simulink model "Adaptive_CT_ur10v"  (R2021b)
settings: Solver=VariableStepAuto  StartTime=0.0  StopTime=15  FixedStep=1e-4  RelTol=1e1
values from neighbouring files (symbols this model uses):
  Kp = [100 0 0 0 0 0 0 250 0 0 0 0 ... (36 elements, 6x6)]    [ACT_workspace.mat]    (also in GuadagniControllore.m = 100 * diag([1 1 2 4 5 5]))
  Kv = [100 0 0 0 0 0 0 100 0 0 0 0 ... (36 elements, 6x6)]    [ACT_workspace.mat]    (also in GuadagniControllore.m = 100 * diag([1 1 3 3 5 5]))
  l1 = 0.1273    [ACT_workspace.mat]
  l2 = -0.612    [ACT_workspace.mat]
  l3 = -0.5723    [ACT_workspace.mat]
  l4 = 0.1639    [ACT_workspace.mat]
  l5 = 0.1157    [ACT_workspace.mat]
  l6 = 0.0922    [ACT_workspace.mat]
  m1 = 7.1    [ACT_workspace.mat]
  m2 = 12.7    [ACT_workspace.mat]
  m3 = 4.27    [ACT_workspace.mat]
  m4 = 2    [ACT_workspace.mat]
  m5 = 2    [ACT_workspace.mat]
  m6 = 0.365    [ACT_workspace.mat]
  q0 = [0 0 0 0 0 0]    [ACT_workspace.mat]
  r = 0.02    [ACT_workspace.mat]
undefined symbols (not defined in the file or in its folder): B, Spline
libraries: roblocks x2, robotcorelib x1, simulink x1
(part 3 of 20)

== matlab function Adaptive_CT_ur10v/CT control/Subsystem/Regressor ==
  data: q input; Y output; qd input; qdd input
function Y = Regressor(q, qd, qdd)
%#codegen

q2 = q(2);
q3 = q(3);
q4 = q(4);
q5 = q(5);
q6 = q(6);
qd1 = qd(1);
qd2 = qd(2);
qd3 = qd(3);
qd4 = qd(4);
qd5 = qd(5);
qd6 = qd(6);
qdd1 = qdd(1);
qdd2 = qdd(2);
qdd3 = qdd(3);
qdd4 = qdd(4);
qdd5 = qdd(5);
qdd6 = qdd(6);


%    This function was generated by the Symbolic Math Toolbox version 9.0.
%    07-Jul-2022 14:08:40

t2 = cos(q2);
t3 = cos(q3);
t4 = cos(q4);
t5 = cos(q5);
t6 = sin(q2);
t7 = sin(q3);
t8 = sin(q4);
t9 = sin(q5);
t10 = q2+q3;
t11 = q2+q5;
t12 = q3+q4;
t13 = q4+q5;
t14 = qdd2+qdd3;
t15 = q2.*2.0;
t16 = q3.*2.0;
t17 = q4.*2.0;
t18 = q5.*2.0;
t19 = qd1.^2;
t20 = qd2.^2;
t21 = qd3.^2;
t22 = qd4.^2;
t23 = qd5.^2;
t41 = -q5;
t51 = qdd1./2.0;
t52 = qdd2./2.0;
t53 = qdd1./4.0;
t54 = qdd3./2.0;
t55 = qdd4./2.0;
t117 = qdd2.*9.22e-2;
t118 = qdd3.*9.22e-2;
t119 = qdd4.*9.22e-2;
t302 = qdd3.*3.451642e-1;
t397 = qdd3.*3.4091378e-1;
t401 = qdd4.*1.338649e-2;
t402 = qdd4.*1.763691e-2;
t466 = qdd2.*3.2752729e-1;
t467 = qdd3.*3.2752729e-1;
t530 = qdd2.*7.0207129e-1;
t24 = cos(t15);
t25 = cos(t18);
t26 = t2.^2;
t27 = sin(t15);
t28 = sin(t18);
t29 = cos(t10);
t30 = cos(t11);
t31 = cos(t12);
t32 = cos(t13);
t33 = q4+t10;
t34 = q5+t10;
t35 = q5+t12;
t36 = qdd4+t14;
t37 = sin(t10);
t38 = sin(t11);
t39 = sin(t12);
t40 = sin(t13);
t42 = -t18;
t46 = t10+t13;
t50 = q2+t10;
t61 = q2+t41;
t62 = q4+t41;
t63 = t10.*2.0;
t66 = t10+t41;
t67 = t12+t41;
t94 = qd1.*qd2.*t2.*t6.*2.0;
t143 = qdd1.*t5.*3.278e-1;
t145 = qdd2.*t8.*1.1446;
t146 = qdd3.*t8.*1.1446;
t156 = qd2.*qd4.*t4.*1.1446;
t157 = qd3.*qd4.*t4.*1.1446;
t158 = qd1.*qd5.*t9.*3.278e-1;
t178 = qdd2.*t5.*1.157e-1;
t179 = qdd3.*t5.*1.157e-1;
t180 = qdd4.*t5.*1.157e-1;
t181 = qdd5.*t5.*1.157e-1;
t184 = qdd4.*t8.*5.723e-1;
t211 = t2.*6.00372;
t248 = t4.*t22.*5.723e-1;
t251 = t9.*t23.*1.157e-1;
t252 = t9.*t19.*1.639e-1;
t348 = qdd1.*t6.*1.003068e-1;
t349 = qdd2.*t6.*1.003068e-1;
t379 = qdd2.*t3.*7.004952e-1;
t380 = qdd1.*t3.*3.502476e-1;
t381 = qdd2.*t3.*3.502476e-1;
t382 = qdd3.*t3.*3.502476e-1;
t418 = t2.*t20.*1.003068e-1;
t422 = qd2.*qd3.*t7.*7.004952e-1;
t423 = qd1.*qd3.*t7.*3.502476e-1;
t454 = qdd5.*t5.*1.066754e-2;
t463 = qdd2.*t8.*1.3243022e-1;
t464 = qdd3.*t8.*1.3243022e-1;
t479 = t7.*t20.*3.502476e-1;
t480 = t7.*t21.*3.502476e-1;
t481 = t7.*t19.*1.751238e-1;
t483 = qd2.*qd3.*t4.*1.3243022e-1;
t484 = qd2.*qd4.*t4.*1.3243022e-1;
t485 = qd3.*qd4.*t4.*1.3243022e-1;
t525 = qdd1.*t8.*6.621511e-2;
t526 = qdd2.*t8.*6.621511e-2;
t527 = qdd3.*t8.*6.621511e-2;
t528 = qdd4.*t8.*6.621511e-2;
t542 = t9.*t23.*1.066754e-2;
t545 = qd1.*qd4.*t4.*6.621511e-2;
t595 = t4.*t20.*6.621511e-2;
t596 = t4.*t21.*6.621511e-2;
t597 = t4.*t22.*6.621511e-2;
t598 = t4.*t19.*3.3107555e-2;
t43 = cos(t33);
t44 = cos(t34);
t45 = cos(t35);
t47 = sin(t33);
t48 = sin(t34);
t49 = sin(t35);
t56 = cos(t50);
t57 = q2+t33;
t58 = sin(t50);
t59 = cos(t46);
t60 = sin(t46);
t64 = cos(t61);
t65 = cos(t62);
t68 = sin(t61);
t69 = sin(t62);
t71 = t13+t34;
t72 = t11+t33;
t74 = qd2.*qd3.*t28;
t75 = qd2.*qd4.*t28;
t76 = qd2.*qd5.*t28;
t77 = qd3.*qd4.*t28;
t78 = qd3.*qd5.*t28;
t79 = qd4.*qd5.*t28;
t80 = cos(t63);
t82 = t10+t33;
t83 = sin(t63);
t84 = cos(t66);
t85 = cos(t67);
t86 = t33+t41;
t87 = t33+t42;
t88 = sin(t66);
t89 = sin(t67);
t95 = t25.*t52;
t96 = t25.*t53;
t97 = t25.*t54;
t98 = t25.*t55;
t103 = t10+t46;
t109 = qdd2.*t25.*(-1.0./2.0);
t110 = qdd3.*t25.*(-1.0./2.0);
t111 = qdd4.*t25.*(-1.0./2.0);
t115 = (qd1.*qd5.*t28)./2.0;
t116 = t17+t63;
t122 = t33+t46;
t126 = (t19.*t27)./2.0;
t127 = (t20.*t28)./2.0;
t128 = (t19.*t28)./4.0;
t129 = (t21.*t28)./2.0;
t130 = (t22.*t28)./2.0;
t133 = t33+t66;
t137 = qdd2.*t39.*(1.53e+2./2.5e+2);
t138 = qdd1.*t38.*(1.53e+2./5.0e+2);
t139 = qdd2.*t38.*(1.53e+2./5.0e+2);
t140 = qdd5.*t38.*(1.53e+2./5.0e+2);
t141 = t46.*2.0;
t152 = t25.*t117;
t153 = t25.*t118;
t154 = t25.*t119;
t182 = -t145;
t183 = -t146;
t190 = qd1.*qd2.*t30.*(1.53e+2./2.5e+2);
t191 = qd1.*qd5.*t30.*(1.53e+2./2.5e+2);
t200 = qdd2.*t25.*(-9.22e-2);
t201 = qdd3.*t25.*(-9.22e-2);
t202 = qdd4.*t25.*(-9.22e-2);
t205 = -t156;
t206 = -t157;
t210 = -t158;
t236 = -t178;
t237 = -t179;
t238 = -t180;
t239 = -t181;
t240 = -t184;
t242 = t20.*t31.*(1.53e+2./2.5e+2);
t243 = t19.*t31.*(1.53e+2./5.0e+2);
t244 = t20.*t30.*(1.53e+2./5.0e+2);
t245 = t23.*t30.*(1.53e+2./5.0e+2);
t256 = -t211;
t263 = qdd2.*t40.*5.723e-1;
t264 = qdd3.*t40.*5.723e-1;
t265 = qdd1.*t40.*2.8615e-1;
t266 = qdd2.*t40.*2.8615e-1;
t267 = qdd3.*t40.*2.8615e-1;
t268 = qdd4.*t40.*2.8615e-1;
t269 = qdd5.*t40.*2.8615e-1;
t279 = -t248;
t307 = qd2.*qd3.*t32.*5.723e-1;
t308 = qd2.*qd4.*t32.*5.723e-1;
t309 = qd2.*qd5.*t32.*5.723e-1;
t310 = qd3.*qd4.*t32.*5.723e-1;
t311 = qd3.*qd5.*t32.*5.723e-1;
t312 = qd4.*qd5.*t32.*5.723e-1;
t313 = qd1.*qd4.*t32.*2.8615e-1;
t314 = qd1.*qd5.*t32.*2.8615e-1;
t319 = qdd1.*t24.*1.87272e-1;
t346 = qd1.*qd2.*t27.*3.74544e-1;
t359 = t20.*t32.*2.8615e-1;
t360 = t21.*t32.*2.8615e-1;
t361 = t22.*t32.*2.8615e-1;
t362 = t23.*t32.*2.8615e-1;
t363 = t19.*t32.*1.43075e-1;
t417 = t29.*5.614263;
t442 = t19.*t27.*1.87272e-1;
t443 = qdd2.*t39.*1.416168e-1;
t444 = qdd1.*t38.*2.82132e-2;
t445 = qdd1.*t39.*7.08084e-2;
t446 = qdd2.*t39.*7.08084e-2;
t447 = qdd3.*t39.*7.08084e-2;
t448 = qdd4.*t39.*7.08084e-2;
t476 = qdd2.*t25.*4.25042e-3;
t477 = qdd3.*t25.*4.25042e-3;
t478 = qdd4.*t25.*4.25042e-3;
t487 = -t422;
t488 = -t423;
t516 = -t454;
t523 = -t463;
t524 = -t464;
t531 = qd2.*qd3.*t31.*1.416168e-1;
t532 = qd2.*qd4.*t31.*1.416168e-1;
t533 = qd3.*qd4.*t31.*1.416168e-1;
t534 = qd1.*qd3.*t31.*7.08084e-2;
t535 = qd1.*qd4.*t31.*7.08084e-2;
t541 = -t480;
t543 = -t484;
t544 = -t485;
t574 = qdd2.*t40.*5.276606e-2;
t575 = qdd3.*t40.*5.276606e-2;
t580 = -t525;
t581 = -t526;
t582 = -t527;
t583 = -t528;
t584 = t20.*t31.*7.08084e-2;
t585 = t21.*t31.*7.08084e-2;
t586 = t22.*t31.*7.08084e-2;
t587 = t19.*t31.*3.54042e-2;
t599 = -t545;
t619 = qdd2.*t40.*2.638303e-2;
t620 = qdd3.*t40.*2.638303e-2;
t621 = qdd4.*t40.*2.638303e-2;
t622 = qdd5.*t40.*2.638303e-2;
t628 = qd2.*qd3.*t32.*5.276606e-2;
t629 = qd2.*qd4.*t32.*5.276606e-2;
t630 = qd2.*qd5.*t32.*5.276606e-2;
t631 = qd3.*qd4.*t32.*5.276606e-2;
t632 = qd3.*qd5.*t32.*5.276606e-2;
t633 = qd4.*qd5.*t32.*5.276606e-2;
t634 = -t597;
t654 = qdd1.*t37.*9.379997e-2;
t655 = qdd2.*t37.*9.379997e-2;
t656 = qdd3.*t37.*9.379997e-2;
t661 = qd2.*qd3.*t29.*1.8759994e-1;
t683 = t20.*t32.*2.638303e-2;
t684 = t21.*t32.*2.638303e-2;
t685 = t22.*t32.*2.638303e-2;
t686 = t23.*t32.*2.638303e-2;
t688 = t19.*t32.*1.3191515e-2;
t713 = t20.*t29.*9.379997e-2;
t714 = t21.*t29.*9.379997e-2;
t70 = cos(t57);
t73 = sin(t57);
t81 = qd1.*qd5.*t47;
t90 = cos(t71);
t91 = cos(t72);
t92 = sin(t71);
t93 = sin(t72);
t99 = -t76;
t100 = -t78;
t101 = -t79;
t102 = cos(t82);
t104 = sin(t82);
t105 = cos(t86);
t106 = cos(t87);
t107 = sin(t86);
t108 = sin(t87);
t112 = cos(t103);
t113 = sin(t103);
t120 = t41+t57;
t121 = cos(t116);
t123 = sin(t116);
t131 = qd1.*qd2.*t83;
t132 = qd1.*qd3.*t83;
t134 = cos(t122);
t135 = sin(t122);
t136 = t51.*t80;
t142 = cos(t133);
t144 = sin(t133);
t151 = cos(t141);
t155 = sin(t141);
t169 = t47.*(9.81e+2./1.0e+2);
t170 = -t137;
t171 = -t138;
t172 = -t140;
t176 = t41+t116;
t177 = t42+t116;
t192 = qdd2.*t49.*(1.53e+2./2.5e+2);
t193 = qdd1.*t49.*(1.53e+2./5.0e+2);
t194 = qdd2.*t49.*(1.53e+2./5.0e+2);
t195 = qdd3.*t49.*(1.53e+2./5.0e+2);
t196 = qdd4.*t49.*(1.53e+2./5.0e+2);
t197 = qdd5.*t49.*(1.53e+2./5.0e+2);
t223 = qd2.*qd3.*t45.*(1.53e+2./2.5e+2);
t224 = qd2.*qd4.*t45.*(1.53e+2./2.5e+2);
t225 = qd2.*qd5.*t45.*(1.53e+2./2.5e+2);
t226 = qd3.*qd4.*t45.*(1.53e+2./2.5e+2);
t227 = qd3.*qd5.*t45.*(1.53e+2./2.5e+2);
t228 = qd4.*qd5.*t45.*(1.53e+2./2.5e+2);
t229 = qd1.*qd3.*t45.*(1.53e+2./5.0e+2);
t230 = qd1.*qd4.*t45.*(1.53e+2./5.0e+2);
t231 = qd1.*qd5.*t45.*(1.53e+2./5.0e+2);
t232 = t76.*1.844e-1;
t233 = t78.*1.844e-1;
t234 = t79.*1.844e-1;
t235 = (t19.*t83)./2.0;
t246 = -t190;
t247 = t60.*(9.81e+2./2.0e+2);
t258 = t20.*t45.*(1.53e+2./5.0e+2);
t259 = t21.*t45.*(1.53e+2./5.0e+2);
t260 = t22.*t45.*(1.53e+2./5.0e+2);
t261 = t23.*t45.*(1.53e+2./5.0e+2);
t274 = -t245;
t275 = qdd1.*t68.*(1.53e+2./5.0e+2);
t276 = qdd2.*t68.*(1.53e+2./5.0e+2);
t277 = qdd5.*t68.*(1.53e+2./5.0e+2);
t282 = t19.*t45.*(1.53e+2./1.0e+3);
t283 = qd1.*qd2.*t64.*(1.53e+2./2.5e+2);
t284 = qd1.*qd5.*t64.*(1.53e+2./2.5e+2);
t285 = qdd2.*t89.*(1.53e+2./2.5e+2);
t286 = qdd1.*t89.*(1.53e+2./5.0e+2);
t287 = qdd2.*t89.*(1.53e+2./5.0e+2);
t288 = qdd3.*t89.*(1.53e+2./5.0e+2);
t289 = qdd4.*t89.*(1.53e+2./5.0e+2);
t290 = qdd5.*t89.*(1.53e+2./5.0e+2);
t291 = qdd1.*t59.*1.398e-1;
t292 = qdd5.*t59.*1.398e-1;
t293 = qdd1.*t59.*2.41e-2;
t294 = qdd2.*t59.*2.41e-2;
t295 = qdd3.*t59.*2.41e-2;
t296 = qdd4.*t59.*2.41e-2;
t303 = qd2.*qd3.*t60.*4.82e-2;
t304 = qd2.*qd4.*t60.*4.82e-2;
t305 = qd3.*qd4.*t60.*4.82e-2;
t306 = qdd1.*t43.*1.639e-1;
t315 = qdd1.*t48.*2.8615e-1;
t316 = qdd2.*t48.*2.8615e-1;
t317 = qdd3.*t48.*2.8615e-1;
t318 = qdd5.*t48.*2.8615e-1;
t324 = t20.*t64.*(1.53e+2./5.0e+2);
t325 = t23.*t64.*(1.53e+2./5.0e+2);
t340 = qd1.*qd2.*t44.*5.723e-1;
t341 = qd1.*qd3.*t44.*5.723e-1;
t342 = qd2.*qd3.*t44.*5.723e-1;
t343 = qd1.*qd5.*t44.*5.723e-1;
t350 = qd2.*qd3.*t85.*(1.53e+2./2.5e+2);
t351 = qd2.*qd4.*t85.*(1.53e+2./2.5e+2);
t352 = qd2.*qd5.*t85.*(1.53e+2./2.5e+2);
t353 = qd3.*qd4.*t85.*(1.53e+2./2.5e+2);
t354 = qd3.*qd5.*t85.*(1.53e+2./2.5e+2);
t355 = qd4.*qd5.*t85.*(1.53e+2./2.5e+2);
t356 = qd1.*qd3.*t85.*(1.53e+2./5.0e+2);
t357 = qd1.*qd4.*t85.*(1.53e+2./5.0e+2);
t358 = qd1.*qd5.*t85.*(1.53e+2./5.0e+2);
t364 = -t307;
t370 = t20.*t44.*2.8615e-1;
t371 = t21.*t44.*2.8615e-1;
t372 = t23.*t44.*2.8615e-1;
t378 = -t346;
t383 = t20.*t85.*(1.53e+2./5.0e+2);
t384 = t21.*t85.*(1.53e+2./5.0e+2);
t385 = t22.*t85.*(1.53e+2./5.0e+2);
t386 = t23.*t85.*(1.53e+2./5.0e+2);
t393 = t23.*t60.*1.398e-1;
t394 = t20.*t60.*2.41e-2;
t395 = t21.*t60.*2.41e-2;
t396 = t22.*t60.*2.41e-2;
t398 = -t359;
t399 = -t360;
t400 = -t363;
t403 = qd1.*qd2.*t60.*1.157e-1;
t404 = qd1.*qd3.*t60.*1.157e-1;
t405 = qd1.*qd4.*t60.*1.157e-1;
t406 = qd1.*qd5.*t60.*1.157e-1;
t407 = qd2.*qd5.*t60.*1.639e-1;
t408 = qd3.*qd5.*t60.*1.639e-1;
t409 = qd4.*qd5.*t60.*1.639e-1;
t410 = qdd2.*t69.*5.723e-1;
t411 = qdd3.*t69.*5.723e-1;
t412 = qdd1.*t69.*2.8615e-1;
t413 = qdd2.*t69.*2.8615e-1;
t414 = qdd3.*t69.*2.8615e-1;
t415 = qdd4.*t69.*2.8615e-1;
t416 = qdd5.*t69.*2.8615e-1;
t426 = qd2.*qd3.*t65.*5.723e-1;
t427 = qd2.*qd4.*t65.*5.723e-1;
t428 = qd2.*qd5.*t65.*5.723e-1;
t429 = qd3.*qd4.*t65.*5.723e-1;
t430 = qd3.*qd5.*t65.*5.723e-1;
t431 = qd4.*qd5.*t65.*5.723e-1;
t432 = qd1.*qd4.*t65.*2.8615e-1;
t433 = qd1.*qd5.*t65.*2.8615e-1;
t434 = qdd1.*t88.*2.8615e-1;
t435 = qdd2.*t88.*2.8615e-1;
t436 = qdd3.*t88.*2.8615e-1;
t437 = qdd5.*t88.*2.8615e-1;
t453 = t19.*t85.*(1.53e+2./1.0e+3);
t475 = -t417;
t489 = t20.*t65.*2.8615e-1;
t490 = t21.*t65.*2.8615e-1;
t491 = t22.*t65.*2.8615e-1;
t492 = t23.*t65.*2.8615e-1;
t493 = t19.*t65.*1.43075e-1;
t505 = t47.*1.135017;
t506 = -t443;
t507 = -t445;
t508 = -t446;
t509 = -t447;
t510 = -t448;
t519 = qd1.*qd2.*t84.*5.723e-1;
t520 = qd1.*qd3.*t84.*5.723e-1;
t521 = qd2.*qd3.*t84.*5.723e-1;
t522 = qd1.*qd5.*t84.*5.723e-1;
t536 = t60.*4.52241e-1;
t537 = qdd2.*t49.*2.82132e-2;
t538 = -t476;
t539 = -t477;
t540 = -t478;
t568 = t76.*8.50084e-3;
t569 = t78.*8.50084e-3;
t570 = t79.*8.50084e-3;
t576 = t20.*t84.*2.8615e-1;
t577 = t21.*t84.*2.8615e-1;
t578 = t23.*t84.*2.8615e-1;
t588 = -t531;
t589 = -t532;
t590 = -t533;
t591 = -t534;
t592 = -t535;
t609 = t20.*t45.*2.82132e-2;
t610 = t19.*t45.*1.41066e-2;
t612 = qdd1.*t59.*2.22202e-3;
t624 = -t585;
t625 = -t586;
t626 = qdd1.*t56.*3.502476e-1;
t627 = qdd1.*t68.*2.82132e-2;
t639 = qdd2.*t89.*2.82132e-2;
t641 = qd1.*qd2.*t58.*7.004952e-1;
t642 = qd1.*qd3.*t58.*3.502476e-1;
t644 = qd1.*qd5.*t44.*5.276606e-2;
t646 = qd2.*qd3.*t47.*3.792646e-2;
t647 = qd2.*qd4.*t47.*3.792646e-2;
t648 = qd3.*qd4.*t47.*3.792646e-2;
t660 = -t628;
t662 = qdd1.*t43.*1.896323e-2;
t663 = qdd2.*t43.*1.896323e-2;
t664 = qdd3.*t43.*1.896323e-2;
t665 = qdd4.*t43.*1.896323e-2;
t666 = qdd1.*t48.*2.638303e-2;
t667 = t19.*t58.*3.502476e-1;
t668 = t19.*t58.*1.751238e-1;
t687 = qd1.*qd5.*t60.*1.066754e-2;
t689 = qdd2.*t69.*5.276606e-2;
t690 = qdd3.*t69.*5.276606e-2;
t697 = qd2.*qd3.*t65.*5.276606e-2;
t698 = qd2.*qd4.*t65.*5.276606e-2;
t699 = qd2.*qd5.*t65.*5.276606e-2;
t700 = qd3.*qd4.*t65.*5.276606e-2;
t701 = qd3.*qd5.*t65.*5.276606e-2;
t702 = qd4.*qd5.*t65.*5.276606e-2;
t703 = t20.*t47.*1.896323e-2;
t704 = t21.*t47.*1.896323e-2;
t705 = t22.*t47.*1.896323e-2;
t707 = t20.*t85.*2.82132e-2;
t708 = t19.*t85.*1.41066e-2;
t711 = -t683;
t712 = -t684;
t716 = -t688;
t725 = qdd2.*t69.*2.638303e-2;
t726 = qdd3.*t69.*2.638303e-2;
t727 = qdd4.*t69.*2.638303e-2;
t728 = qdd5.*t69.*2.638303e-2;
t741 = qdd1.*t88.*2.638303e-2;
t742 = qd1.*qd5.*t84.*5.276606e-2;
t754 = t20.*t65.*2.638303e-2;
t755 = t21.*t65.*2.638303e-2;
t756 = t22.*t65.*2.638303e-2;
t757 = t23.*t65.*2.638303e-2;
t759 = t19.*t65.*1.3191515e-2;
t760 = qdd1.*t80.*1.63763645e-1;
t789 = t19.*t83.*1.63763645e-1;
t114 = -t81;
t124 = cos(t120);
t125 = sin(t120);
t147 = t53.*t90;
t148 = (qdd2.*t90)./4.0;
t149 = (qdd3.*t90)./4.0;
Y = ft_1({qd1,qd2,qd3,qd4,qd5,qdd1,qdd2,qdd3,qdd4,qdd5,t100,t101,t102,t104,t105,t106,t107,t108,t109,t110,t111,t112,t113,t114,t115,t117,t118,t119,t121,t123,t124,t125,t126,t127,t128,t129,t130,t131,t132,t134,t135,t136,t138,t139,t14,t142,t143,t144,t147,t148,t149,t151,t155,t169,t170,t171,t172,t176,t177,t182,t183,t19,t191,t192,t193,t194,t195,t196,t197,t2,t20,t200,t201,t202,t205,t206,t21,t210,t22,t223,t224,t225,t226,t227,t228,t229,t23,t230,t231,t232,t233,t234,t235,t236,t237,t238,t239,t240,t242,t243,t244,t246,t247,t25,t251,t252,t256,t258,t259,t26,t260,t261,t263,t264,t265,t266,t267,t268,t269,t274,t275,t276,t277,t279,t28,t282,t283,t284,t285,t286,t287,t288,t289,t290,t291,t292,t293,t294,t295,t296,t30,t302,t303,t304,t305,t306,t308,t309,t31,t310,t311,t312,t313,t314,t315,t316,t317,t318,t319,t32,t324,t325,t340,t341,t342,t343,t348,t349,t350,t351,t352,t353,t354,t355,t356,t357,t358,t36,t361,t362,t364,t370,t371,t372,t378,t379,t38,t380,t381,t382,t383,t384,t385,t386,t39,t393,t394,t395,t396,t397,t398,t399,t4,t40,t400,t401,t402,t403,t404,t405,t406,t407,t408,t409,t410,t411,t412,t413,t414,t415,t416,t418,t426,t427,t428,t429,t43,t430,t431,t432,t433,t434,t435,t436,t437,t44,t442,t444,t45,t453,t466,t467,t47,t475,t479,t48,t481,t483,t487,t488,t489,t49,t490,t491,t492,t493,t5,t505,t506,t507,t508,t509,t51,t510,t516,t519,t52,t520,t521,t522,t523,t524,t53,t530,t536,t537,t538,t539,t54,t540,t541,t542,t543,t544,t55,t568,t569,t570,t574,t575,t576,t577,t578,t580,t581,t582,t583,t584,t587,t588,t589,t59,t590,t591,t592,t595,t596,t598,t599,t6,t60,t609,t610,t612,t619,t620,t621,t622,t624,t625,t626,t627,t629,t630,t631,t632,t633,t634,t639,t64,t641,t642,t644,t646,t647,t648,t65,t654,t655,t656,t660,t661,t662,t663,t664,t665,t666,t667,t668,t68,t685,t686,t687,t689,t69,t690,t697,t698,t699,t70,t700,t701,t702,t703,t704,t705,t707,t708,t711,t712,t713,t714,t716,t725,t726,t727,t728,t73,t74,t741,t742,t75,t754,t755,t756,t757,t759,t76,t760,t77,t78,t789,t79,t8,t80,t81,t84,t85,t88,t89,t9,t90,t91,t92,t93,t94,t95,t96,t97,t98,t99});
end
function Y = ft_1(ct)
qd1 = ct{1};
qd2 = ct{2};
qd3 = ct{3};
qd4 = ct{4};
qd5 = ct{5};
qdd1 = ct{6};
qdd2 = ct{7};
qdd3 = ct{8};
qdd4 = ct{9};
qdd5 = ct{10};
t100 = ct{11};
t101 = ct{12};
t102 = ct{13};
t104 = ct{14};
t105 = ct{15};
t106 = ct{16};
t107 = ct{17};
t108 = ct{18};
t109 = ct{19};
t110 = ct{20};
t111 = ct{21};
t112 = ct{22};
t113 = ct{23};
t114 = ct{24};
t115 = ct{25};
t117 = ct{26};
t118 = ct{27};
t119 = ct{28};
t121 = ct{29};
t123 = ct{30};
t124 = ct{31};
t125 = ct{32};
t126 = ct{33};
t127 = ct{34};
t128 = ct{35};
t129 = ct{36};
t130 = ct{37};
t131 = ct{38};
t132 = ct{39};
t134 = ct{40};
t135 = ct{41};
t136 = ct{42};
t138 = ct{43};
t139 = ct{44};
t14 = ct{45};
t142 = ct{46};
t143 = ct{47};
t144 = ct{48};
t147 = ct{49};
t148 = ct{50};
t149 = ct{51};
t151 = ct{52};
t155 = ct{53};
t169 = ct{54};
t170 = ct{55};
t171 = ct{56};
t172 = ct{57};
t176 = ct{58};
t177 = ct{59};
t182 = ct{60};
t183 = ct{61};
t19 = ct{62};
t191 = ct{63};
t192 = ct{64};
t193 = ct{65};
t194 = ct{66};
t195 = ct{67};
t196 = ct{68};
t197 = ct{69};
t2 = ct{70};
t20 = ct{71};
t200 = ct{72};
t201 = ct{73};
t202 = ct{74};
t205 = ct{75};
t206 = ct{76};
t21 = ct{77};
t210 = ct{78};
t22 = ct{79};
t223 = ct{80};
t224 = ct{81};
t225 = ct{82};
t226 = ct{83};
t227 = ct{84};
t228 = ct{85};
t229 = ct{86};
t23 = ct{87};
t230 = ct{88};
t231 = ct{89};
t232 = ct{90};
t233 = ct{91};
t234 = ct{92};
t235 = ct{93};
t236 = ct{94};
t237 = ct{95};
t238 = ct{96};
t239 = ct{97};
t240 = ct{98};
t242 = ct{99};
t243 = ct{100};
t244 = ct{101};
t246 = ct{102};
t247 = ct{103};
t25 = ct{104};
t251 = ct{105};
t252 = ct{106};
t256 = ct{107};
t258 = ct{108};
t259 = ct{109};
t26 = ct{110};
t260 = ct{111};
t261 = ct{112};
t263 = ct{113};
t264 = ct{114};
t265 = ct{115};
t266 = ct{116};
t267 = ct{117};
t268 = ct{118};
t269 = ct{119};
t274 = ct{120};
t275 = ct{121};
t276 = ct{122};
t277 = ct{123};
t279 = ct{124};
t28 = ct{125};
t282 = ct{126};
t283 = ct{127};
t284 = ct{128};
t285 = ct{129};
t286 = ct{130};
t287 = ct{131};
t288 = ct{132};
t289 = ct{133};
t290 = ct{134};
t291 = ct{135};
t292 = ct{136};
t293 = ct{137};
t294 = ct{138};
t295 = ct{139};
t296 = ct{140};
t30 = ct{141};
t302 = ct{142};
t303 = ct{143};
t304 = ct{144};
t305 = ct{145};
t306 = ct{146};
t308 = ct{147};
t309 = ct{148};
t31 = ct{149};
t310 = ct{150};
t311 = ct{151};
t312 = ct{152};
t313 = ct{153};
t314 = ct{154};
t315 = ct{155};
t316 = ct{156};
t317 = ct{157};
t318 = ct{158};
t319 = ct{159};
t32 = ct{160};
t324 = ct{161};
t325 = ct{162};
t340 = ct{163};
t341 = ct{164};
t342 = ct{165};
t343 = ct{166};
t348 = ct{167};
t349 = ct{168};
t350 = ct{169};
t351 = ct{170};
t352 = ct{171};
t353 = ct{172};
t354 = ct{173};
t355 = ct{174};
t356 = ct{175};
t357 = ct{176};
t358 = ct{177};
t36 = ct{178};
t361 = ct{179};
t362 = ct{180};
t364 = ct{181};
t370 = ct{182};
t371 = ct{183};
t372 = ct{184};
t378 = ct{185};
t379 = ct{186};
t38 = ct{187};
t380 = ct{188};
t381 = ct{189};
t382 = ct{190};
t383 = ct{191};
t384 = ct{192};
t385 = ct{193};
t386 = ct{194};
t39 = ct{195};
t393 = ct{196};
t394 = ct{197};
t395 = ct{198};
t396 = ct{199};
t397 = ct{200};
t398 = ct{201};
t399 = ct{202};
t4 = ct{203};
t40 = ct{204};
t400 = ct{205};
t401 = ct{206};
t402 = ct{207};
t403 = ct{208};
t404 = ct{209};
t405 = ct{210};
t406 = ct{211};
t407 = ct{212};
t408 = ct{213};
t409 = ct{214};
t410 = ct{215};
t411 = ct{216};
t412 = ct{217};
t413 = ct{218};
t414 = ct{219};
t415 = ct{220};
t416 = ct{221};
t418 = ct{222};
t426 = ct{223};
t427 = ct{224};
t428 = ct{225};
t429 = ct{226};
t43 = ct{227};
t430 = ct{228};
t431 = ct{229};
t432 = ct{230};
t433 = ct{231};
t434 = ct{232};
t435 = ct{233};
t436 = ct{234};
t437 = ct{235};
t44 = ct{236};
t442 = ct{237};
t444 = ct{238};
t45 = ct{239};
t453 = ct{240};
t466 = ct{241};
t467 = ct{242};
t47 = ct{243};
t475 = ct{244};
t479 = ct{245};
t48 = ct{246};
t481 = ct{247};
t483 = ct{248};
t487 = ct{249};
t488 = ct{250};
t489 = ct{251};
t49 = ct{252};
t490 = ct{253};
t491 = ct{254};
t492 = ct{255};
t493 = ct{256};
t5 = ct{257};
t505 = ct{258};
t506 = ct{259};
t507 = ct{260};
t508 = ct{261};
t509 = ct{262};
t51 = ct{263};
t510 = ct{264};
t516 = ct{265};
t519 = ct{266};
t52 = ct{267};
t520 = ct{268};
t521 = ct{269};
t522 = ct{270};
t523 = ct{271};
t524 = ct{272};
t53 = ct{273};
t530 = ct{274};
t536 = ct{275};
t537 = ct{276};
t538 = ct{277};
t539 = ct{278};
t54 = ct{279};
t540 = ct{280};
t541 = ct{281};
t542 = ct{282};
t543 = ct{283};
t544 = ct{284};
t55 = ct{285};
t568 = ct{286};
t569 = ct{287};
t570 = ct{288};
t574 = ct{289};
t575 = ct{290};
t576 = ct{291};
t577 = ct{292};
t578 = ct{293};
t580 = ct{294};
t581 = ct{295};
t582 = ct{296};
t583 = ct{297};
t584 = ct{298};
t587 = ct{299};
t588 = ct{300};
t589 = ct{301};
t59 = ct{302};
t590 = ct{303};
t591 = ct{304};
t592 = ct{305};
t595 = ct{306};
t596 = ct{307};
t598 = ct{308};
t599 = ct{309};
t6 = ct{310};
t60 = ct{311};
t609 = ct{312};
t610 = ct{313};
t612 = ct{314};
t619 = ct{315};
t620 = ct{316};
t621 = ct{317};
t622 = ct{318};
t624 = ct{319};
t625 = ct{320};
t626 = ct{321};
t627 = ct{322};
t629 = ct{323};
t630 = ct{324};
t631 = ct{325};
t632 = ct{326};
t633 = ct{327};
t634 = ct{328};
t639 = ct{329};
t64 = ct{330};
t641 = ct{331};
t642 = ct{332};
t644 = ct{333};
t646 = ct{334};
t647 = ct{335};
t648 = ct{336};
t65 = ct{337};
t654 = ct{338};
t655 = ct{339};
t656 = ct{340};
t660 = ct{341};
t661 = ct{342};
t662 = ct{343};
t663 = ct{344};
t664 = ct{345};
t665 = ct{346};
t666 = ct{347};
t667 = ct{348};
t668 = ct{349};
t68 = ct{350};
t685 = ct{351};
t686 = ct{352};
t687 = ct{353};
t689 = ct{354};
t69 = ct{355};
t690 = ct{356};
t697 = ct{357};
t698 = ct{358};
t699 = ct{359};
t70 = ct{360};
t700 = ct{361};
t701 = ct{362};
t702 = ct{363};
t703 = ct{364};
t704 = ct{365};
t705 = ct{366};
t707 = ct{367};
t708 = ct{368};
t711 = ct{369};
t712 = ct{370};
t713 = ct{371};
t714 = ct{372};
t716 = ct{373};
t725 = ct{374};
t726 = ct{375};
t727 = ct{376};
t728 = ct{377};
t73 = ct{378};
t74 = ct{379};
t741 = ct{380};
t742 = ct{381};
t75 = ct{382};
t754 = ct{383};
t755 = ct{384};
t756 = ct{385};
t757 = ct{386};
t759 = ct{387};
t76 = ct{388};
t760 = ct{389};
t77 = ct{390};
t78 = ct{391};
t789 = ct{392};
t79 = ct{393};
t8 = ct{394};
t80 = ct{395};
t81 = ct{396};
t84 = ct{397};
t85 = ct{398};
t88 = ct{399};
t89 = ct{400};
t9 = ct{401};
t90 = ct{402};
t91 = ct{403};
t92 = ct{404};
t93 = ct{405};
t94 = ct{406};
t95 = ct{407};
t96 = ct{408};
t97 = ct{409};
t98 = ct{410};
t99 = ct{411};
t150 = (qdd4.*t90)./4.0;
t159 = (qd1.*qd2.*t92)./2.0;
t160 = (qd1.*qd3.*t92)./2.0;
t161 = (qd1.*qd4.*t92)./2.0;
t162 = (qd2.*qd3.*t92)./2.0;
t163 = (qd1.*qd5.*t92)./2.0;
t164 = (qd2.*qd4.*t92)./2.0;
t165 = (qd2.*qd5.*t92)./2.0;
t166 = (qd3.*qd4.*t92)./2.0;
t167 = (qd3.*qd5.*t92)./2.0;
t168 = (qd4.*qd5.*t92)./2.0;
t173 = qd1.*qd2.*t123;
t174 = qd1.*qd3.*t123;
t175 = qd1.*qd4.*t123;
t185 = t53.*t106;
t186 = qdd1.*t90.*(-1.0./4.0);
t187 = (qdd2.*t106)./4.0;
t188 = (qdd3.*t106)./4.0;
t189 = (qdd4.*t106)./4.0;
t198 = cos(t176);
t199 = cos(t177);
t203 = sin(t176);
t204 = sin(t177);
t207 = (t20.*t92)./4.0;
t208 = (t21.*t92)./4.0;
t209 = (t22.*t92)./4.0;
t212 = (qd1.*qd2.*t108)./2.0;
t213 = (qd1.*qd3.*t108)./2.0;
t214 = (qd1.*qd4.*t108)./2.0;
t215 = (qd2.*qd3.*t108)./2.0;
t216 = (qd1.*qd5.*t108)./2.0;
t218 = (qd2.*qd4.*t108)./2.0;
t219 = (qd2.*qd5.*t108)./2.0;
t220 = (qd3.*qd4.*t108)./2.0;
t221 = (qd3.*qd5.*t108)./2.0;
t222 = (qd4.*qd5.*t108)./2.0;
t241 = qdd1.*t106.*(-1.0./4.0);
t249 = t51.*t121;
t250 = t53.*t121;
t253 = (t20.*t108)./4.0;
t254 = (t21.*t108)./4.0;
t255 = (t22.*t108)./4.0;
t262 = t81.*1.844e-1;
t273 = -t235;
t278 = -t247;
t280 = qdd1.*t121.*(-1.0./4.0);
t281 = -t258;
t301 = qdd1.*t93.*(1.53e+2./5.0e+2);
t320 = qd1.*qd2.*t91.*(1.53e+2./2.5e+2);
t321 = qd1.*qd3.*t91.*(1.53e+2./5.0e+2);
t322 = qd1.*qd4.*t91.*(1.53e+2./5.0e+2);
t323 = qd1.*qd5.*t91.*(1.53e+2./5.0e+2);
t326 = -t282;
t327 = -t284;
t328 = t107.*(9.81e+2./2.0e+2);
t329 = -t285;
t330 = -t286;
t331 = -t287;
t332 = -t288;
t333 = -t289;
t334 = -t291;
t335 = -t292;
t336 = -t293;
t337 = -t294;
t338 = -t295;
t339 = -t296;
t344 = (t19.*t123)./2.0;
t345 = (t19.*t123)./4.0;
t347 = t19.*t70.*(1.53e+2./5.0e+2);
t365 = -t315;
t366 = -t318;
t367 = t19.*t91.*(1.53e+2./5.0e+2);
t368 = -t325;
t369 = qd1.*qd5.*t92.*9.22e-2;
t374 = -t340;
t375 = -t341;
t387 = qdd1.*t90.*4.61e-2;
t388 = -t350;
t389 = -t351;
t390 = -t353;
t391 = -t356;
t392 = -t357;
t420 = t19.*t91.*(1.53e+2./1.0e+3);
t424 = qd1.*qd5.*t108.*9.22e-2;
t425 = -t372;
t438 = (qd1.*qd2.*t155)./4.0;
t439 = (qd1.*qd3.*t155)./4.0;
t440 = (qd1.*qd4.*t155)./4.0;
t441 = (qd1.*qd5.*t155)./4.0;
t449 = -t383;
t450 = -t384;
t451 = -t385;
t452 = -t386;
t455 = qdd1.*t105.*1.398e-1;
t456 = qdd2.*t105.*1.398e-1;
t457 = qdd3.*t105.*1.398e-1;
t458 = qdd4.*t105.*1.398e-1;
t459 = qdd1.*t105.*2.41e-2;
t460 = qdd5.*t105.*2.41e-2;
t461 = qdd1.*t106.*4.61e-2;
t465 = (qdd1.*t151)./8.0;
t468 = -t406;
t469 = -t410;
t470 = -t411;
t471 = -t412;
t472 = -t413;
t473 = -t414;
t474 = -t415;
t494 = qd2.*qd3.*t107.*2.796e-1;
t495 = qd2.*qd4.*t107.*2.796e-1;
t496 = qd3.*qd4.*t107.*2.796e-1;
t497 = -t426;
t498 = -t427;
t499 = -t429;
t500 = -t432;
t515 = -t453;
t546 = qdd1.*t113.*2.8615e-1;
t547 = t20.*t107.*1.398e-1;
t548 = t21.*t107.*1.398e-1;
t549 = t22.*t107.*1.398e-1;
t550 = t23.*t107.*2.41e-2;
t551 = -t489;
t552 = -t490;
t553 = -t491;
t554 = -t492;
t555 = -t493;
t559 = qd1.*qd2.*t107.*1.157e-1;
t560 = qd1.*qd3.*t107.*1.157e-1;
t561 = qd1.*qd4.*t107.*1.157e-1;
t562 = qd1.*qd5.*t107.*1.157e-1;
t563 = qd2.*qd5.*t107.*1.639e-1;
t564 = qd3.*qd5.*t107.*1.639e-1;
t565 = qd4.*qd5.*t107.*1.639e-1;
t566 = (t19.*t155)./8.0;
t579 = -t522;
t593 = -t536;
t594 = t19.*t102.*5.723e-1;
t611 = qdd1.*t73.*7.08084e-2;
t613 = t81.*8.50084e-3;
t615 = qd1.*qd2.*t112.*5.723e-1;
t616 = qd1.*qd3.*t112.*5.723e-1;
t617 = qd1.*qd4.*t112.*2.8615e-1;
t618 = qd1.*qd5.*t112.*2.8615e-1;
t623 = -t578;
t636 = -t609;
t637 = -t610;
t638 = t107.*4.52241e-1;
t643 = -t612;
t649 = t19.*t123.*4.61e-2;
t650 = qdd1.*t134.*5.785e-2;
t652 = t19.*t112.*2.8615e-1;
t653 = t19.*t112.*1.43075e-1;
t657 = qd1.*qd2.*t70.*1.416168e-1;
t658 = qd1.*qd3.*t70.*7.08084e-2;
t659 = qd1.*qd4.*t70.*7.08084e-2;
t669 = -t639;
t670 = -t641;
t671 = -t642;
t672 = -t646;
t673 = -t647;
t674 = -t648;
t677 = qdd1.*t144.*2.8615e-1;
t678 = t19.*t70.*7.08084e-2;
t679 = t19.*t70.*3.54042e-2;
t691 = qd1.*qd2.*t135.*1.157e-1;
t692 = qd1.*qd3.*t135.*1.157e-1;
t693 = qd1.*qd4.*t135.*1.157e-1;
t694 = qd1.*qd5.*t135.*5.785e-2;
t695 = t19.*t91.*1.41066e-2;
t696 = qd1.*qd5.*t92.*4.25042e-3;
t709 = qdd1.*t105.*1.288956e-2;
t710 = qdd1.*t90.*2.12521e-3;
t715 = -t687;
t717 = t19.*t135.*5.785e-2;
t718 = t19.*t135.*2.8925e-2;
t719 = qd1.*qd2.*t142.*5.723e-1;
t720 = qd1.*qd3.*t142.*5.723e-1;
t721 = qd1.*qd4.*t142.*2.8615e-1;
t722 = qd1.*qd5.*t142.*2.8615e-1;
t723 = -t689;
t724 = -t690;
t734 = qd1.*qd5.*t108.*4.25042e-3;
t735 = t19.*t155.*2.305e-2;
t736 = -t698;
t737 = -t700;
t738 = -t703;
t739 = -t704;
t740 = -t705;
t743 = qdd1.*t106.*2.12521e-3;
t746 = t19.*t142.*2.8615e-1;
t747 = t19.*t142.*1.43075e-1;
t751 = -t727;
t752 = qd1.*qd2.*t102.*1.3243022e-1;
t753 = qd1.*qd3.*t102.*1.3243022e-1;
t758 = qd1.*qd5.*t107.*1.066754e-2;
t767 = -t742;
t768 = qdd1.*t104.*6.621511e-2;
t773 = qd1.*qd4.*t102.*6.621511e-2;
t774 = -t756;
t775 = -t757;
t783 = t131.*3.2752729e-1;
t784 = t132.*3.2752729e-1;
t785 = t19.*t102.*6.621511e-2;
t786 = t19.*t102.*3.3107555e-2;
t792 = t19.*t112.*2.638303e-2;
t793 = t19.*t112.*1.3191515e-2;
t795 = t19.*t123.*4.568035e-3;
t796 = t19.*t123.*6.693245e-3;
t800 = t19.*t135.*5.33377e-3;
t801 = t19.*t155.*1.062605e-3;
t802 = t19.*t142.*2.638303e-2;
t803 = t19.*t142.*1.3191515e-2;
t217 = -t163;
t257 = -t216;
t270 = -t173;
t271 = -t174;
t272 = -t175;
t297 = -t262;
t298 = t173./2.0;
t299 = t174./2.0;
t300 = t175./2.0;
t373 = -t328;
t376 = -t344;
t377 = -t345;
t419 = -t367;
t421 = qdd1.*t125.*(1.53e+2./5.0e+2);
t462 = -t387;
t482 = -t420;
t501 = (qd1.*qd2.*t204)./4.0;
t502 = (qd1.*qd3.*t204)./4.0;
t503 = (qd1.*qd4.*t204)./4.0;
t504 = (qd1.*qd5.*t204)./4.0;
t511 = qd1.*qd2.*t124.*(1.53e+2./2.5e+2);
t512 = qd1.*qd3.*t124.*(1.53e+2./5.0e+2);
t513 = qd1.*qd4.*t124.*(1.53e+2./5.0e+2);
t514 = qd1.*qd5.*t124.*(1.53e+2./5.0e+2);
t517 = -t459;
t518 = -t460;
t529 = (qdd1.*t199)./8.0;
t556 = -t494;
t557 = -t495;
t558 = -t496;
t567 = t19.*t124.*(1.53e+2./5.0e+2);
t600 = -t547;
t601 = -t548;
t602 = -t549;
t603 = -t550;
t604 = -t559;
t605 = -t560;
t606 = -t561;
t607 = (t19.*t204)./8.0;
t608 = -t566;
t614 = t19.*t124.*(1.53e+2./1.0e+3);
t640 = -t611;
t645 = -t613;
t675 = -t652;
t676 = -t653;
t680 = -t657;
t681 = -t658;
t682 = -t659;
t706 = -t677;
t729 = -t691;
t730 = -t692;
t731 = -t693;
t732 = -t694;
t733 = -t695;
t744 = -t710;
t745 = qdd1.*t198.*5.785e-2;
t748 = -t719;
t749 = -t720;
t750 = -t721;
t761 = t19.*t204.*2.305e-2;
t762 = -t735;
t763 = qd1.*qd2.*t203.*1.157e-1;
t764 = qd1.*qd3.*t203.*1.157e-1;
t765 = qd1.*qd4.*t203.*1.157e-1;
t766 = qd1.*qd5.*t203.*5.785e-2;
t770 = -t747;
t771 = -t752;
t772 = -t753;
t776 = t114+t344;
t778 = t19.*t203.*5.785e-2;
t779 = t19.*t203.*2.8925e-2;
t781 = t19.*t124.*1.41066e-2;
t782 = -t768;
t787 = -t773;
t790 = -t783;
t791 = -t784;
t794 = -t792;
t797 = -t793;
t798 = -t795;
t799 = -t796;
t804 = t19.*t204.*1.062605e-3;
t805 = -t801;
t806 = t19.*t203.*5.33377e-3;
t486 = -t421;
t571 = -t511;
t572 = -t512;
t573 = -t513;
t635 = -t607;
t651 = -t614;
t769 = -t745;
t777 = -t761;
t780 = -t766;
t788 = -t778;
t807 = -t804;
t808 = -t806;
t810 = t52+t54+t55+t95+t97+t98+t99+t100+t101+t147+t217+t241+t257+t377+t566+t607;
t809 = t52+t54+t55+t76+t78+t79+t109+t110+t111+t163+t185+t186+t216+t377+t608+t635;
et1 = qdd1.*t8.*(-5.723e-1)-qdd1.*t39.*(1.53e+2./2.5e+2)+qdd2.*t43.*1.639e-1+qdd3.*t43.*1.639e-1+qdd4.*t43.*1.639e-1-qdd1.*t73.*(1.53e+2./2.5e+2)-qdd1.*t104.*5.723e-1-t20.*t47.*1.639e-1-t21.*t47.*1.639e-1-t22.*t47.*1.639e-1-qd1.*qd4.*t4.*5.723e-1-qd1.*qd3.*t31.*(1.53e+2./2.5e+2)-qd1.*qd4.*t31.*(1.53e+2./2.5e+2)-qd2.*qd3.*t47.*3.278e-1-qd2.*qd4.*t47.*3.278e-1;
et2 = qd3.*qd4.*t47.*(-3.278e-1)-qd1.*qd2.*t70.*(1.53e+2./1.25e+2)-qd1.*qd3.*t70.*(1.53e+2./2.5e+2)-qd1.*qd4.*t70.*(1.53e+2./2.5e+2)-qd1.*qd2.*t102.*1.1446-qd1.*qd3.*t102.*1.1446-qd1.*qd4.*t102.*5.723e-1;
et3 = qdd1.*3.9096773e-1+t173.*9.13607e-3+t174.*9.13607e-3+t175.*9.13607e-3+t319+t349+t378+t380+t418+t488+t507+t580+t591+t592+t599+t626+t640+t655+t656+t661+t663+t664+t665+t670+t671+t672+t673+t674+t680+t681+t682+t713+t714+t738+t739+t740+t760+t771+t772+t782+t787+t790+t791+qdd1.*t5.*3.022316e-2+qdd1.*t25.*2.12521e-3+qdd2.*t38.*2.82132e-2+qdd1.*t40.*2.638303e-2;
et4 = qdd5.*t38.*(-2.82132e-2)-qdd5.*t43.*8.50084e-3+qdd1.*t49.*2.82132e-2+qdd2.*t48.*2.638303e-2+qdd3.*t48.*2.638303e-2-qdd5.*t48.*2.638303e-2-qdd2.*t59.*2.22202e-3-qdd3.*t59.*2.22202e-3-qdd4.*t59.*2.22202e-3-qdd5.*t59.*1.288956e-2;
et5 = qdd1.*t69.*(-2.638303e-2)+qdd2.*t68.*2.82132e-2+qdd5.*t68.*2.82132e-2-qdd1.*t89.*2.82132e-2+qdd2.*t88.*2.638303e-2+qdd3.*t88.*2.638303e-2-qdd2.*t90.*2.12521e-3-qdd3.*t90.*2.12521e-3+qdd5.*t88.*2.638303e-2+qdd1.*t93.*2.82132e-2;
et6 = qdd4.*t90.*(-2.12521e-3)+qdd2.*t105.*1.288956e-2+qdd2.*t106.*2.12521e-3+qdd3.*t105.*1.288956e-2+qdd3.*t106.*2.12521e-3+qdd4.*t105.*1.288956e-2+qdd4.*t106.*2.12521e-3-qdd5.*t105.*2.22202e-3+qdd1.*t113.*2.638303e-2-qdd1.*t121.*4.568035e-3;
et7 = qdd1.*t125.*(-2.82132e-2)+qdd1.*t134.*5.33377e-3-qdd1.*t144.*2.638303e-2-qdd1.*t151.*1.062605e-3-qdd1.*t198.*5.33377e-3-qdd1.*t199.*1.062605e-3+t20.*t30.*2.82132e-2-t23.*t30.*2.82132e-2+t20.*t44.*2.638303e-2+t21.*t44.*2.638303e-2;
et8 = t23.*t44.*(-2.638303e-2)+t20.*t60.*2.22202e-3+t21.*t60.*2.22202e-3+t22.*t60.*2.22202e-3+t23.*t60.*1.288956e-2+t20.*t64.*2.82132e-2-t23.*t64.*2.82132e-2+t20.*t84.*2.638303e-2+t21.*t84.*2.638303e-2-t23.*t84.*2.638303e-2;
et9 = t20.*t92.*2.12521e-3+t21.*t92.*2.12521e-3+t22.*t92.*2.12521e-3-t20.*t107.*1.288956e-2-t20.*t108.*2.12521e-3-t21.*t107.*1.288956e-2-t21.*t108.*2.12521e-3-t22.*t107.*1.288956e-2-t22.*t108.*2.12521e-3-t23.*t107.*2.22202e-3;
et10 = qd1.*qd5.*t9.*(-3.022316e-2)-qd1.*qd5.*t28.*4.25042e-3+qd1.*qd4.*t32.*2.638303e-2+qd1.*qd5.*t32.*2.638303e-2+qd1.*qd3.*t45.*2.82132e-2+qd2.*qd3.*t44.*5.276606e-2+qd1.*qd4.*t45.*2.82132e-2+qd1.*qd5.*t45.*2.82132e-2+qd2.*qd5.*t47.*8.50084e-3+qd3.*qd5.*t47.*8.50084e-3;
et11 = qd4.*qd5.*t47.*8.50084e-3+qd2.*qd3.*t60.*4.44404e-3+qd2.*qd4.*t60.*4.44404e-3+qd2.*qd5.*t60.*1.511158e-2+qd3.*qd4.*t60.*4.44404e-3+qd3.*qd5.*t60.*1.511158e-2+qd4.*qd5.*t60.*1.511158e-2-qd1.*qd4.*t65.*2.638303e-2+qd1.*qd5.*t65.*2.638303e-2-qd1.*qd3.*t85.*2.82132e-2;
et12 = qd2.*qd3.*t84.*5.276606e-2-qd1.*qd4.*t85.*2.82132e-2+qd1.*qd5.*t85.*2.82132e-2+qd1.*qd2.*t91.*5.64264e-2+qd1.*qd3.*t91.*2.82132e-2+qd1.*qd4.*t91.*2.82132e-2+qd1.*qd5.*t91.*2.82132e-2+qd2.*qd3.*t92.*4.25042e-3+qd2.*qd4.*t92.*4.25042e-3+qd2.*qd5.*t92.*4.25042e-3;
et13 = qd3.*qd4.*t92.*4.25042e-3+qd3.*qd5.*t92.*4.25042e-3+qd4.*qd5.*t92.*4.25042e-3-qd2.*qd3.*t107.*2.577912e-2-qd2.*qd3.*t108.*4.25042e-3-qd2.*qd4.*t107.*2.577912e-2-qd2.*qd4.*t108.*4.25042e-3+qd2.*qd5.*t107.*1.511158e-2-qd3.*qd4.*t107.*2.577912e-2+qd1.*qd2.*t112.*5.276606e-2;
et14 = qd2.*qd5.*t108.*4.25042e-3-qd3.*qd4.*t108.*4.25042e-3+qd3.*qd5.*t107.*1.511158e-2+qd1.*qd3.*t112.*5.276606e-2+qd3.*qd5.*t108.*4.25042e-3+qd4.*qd5.*t107.*1.511158e-2+qd1.*qd4.*t112.*2.638303e-2+qd4.*qd5.*t108.*4.25042e-3+qd1.*qd5.*t112.*2.638303e-2-qd1.*qd2.*t124.*5.64264e-2;
et15 = qd1.*qd3.*t124.*(-2.82132e-2)-qd1.*qd4.*t124.*2.82132e-2+qd1.*qd5.*t124.*2.82132e-2-qd1.*qd2.*t135.*1.066754e-2-qd1.*qd3.*t135.*1.066754e-2-qd1.*qd4.*t135.*1.066754e-2-qd1.*qd5.*t135.*5.33377e-3-qd1.*qd2.*t142.*5.276606e-2-qd1.*qd3.*t142.*5.276606e-2;
et16 = qd1.*qd4.*t142.*(-2.638303e-2)+qd1.*qd5.*t142.*2.638303e-2+qd1.*qd2.*t155.*2.12521e-3+qd1.*qd3.*t155.*2.12521e-3+qd1.*qd4.*t155.*2.12521e-3+qd1.*qd5.*t155.*2.12521e-3+qd1.*qd2.*t203.*1.066754e-2+qd1.*qd2.*t204.*2.12521e-3+qd1.*qd3.*t203.*1.066754e-2;
et17 = qd1.*qd3.*t204.*2.12521e-3+qd1.*qd4.*t203.*1.066754e-2+qd1.*qd4.*t204.*2.12521e-3-qd1.*qd5.*t203.*5.33377e-3-qd1.*qd5.*t204.*2.12521e-3;
et18 = qdd1.*1.383e-1+t139+t143+t172-t173.*9.22e-2-t174.*9.22e-2-t175.*9.22e-2+t193+t210+t229+t230+t231+t244+t265+t274+t276+t277+t301+t303+t304+t305+t313+t314+t316+t317+t320+t321+t322+t323+t324+t330+t335+t337+t338+t339+t342+t358+t366+t368+t370+t371+t391+t392+t393+t394+t395+t396+t407+t408+t409+t425+t433+t435+t436+t437+t456+t457+t458+t471+t486+t500+t514+t518+t521+t546+t556+t557+t558+t563+t564+t565+t571+t572+t573+t576+t577+t600+t601+t602+t603+t615+t616+t617+t618+t623+t650+t706+t722+t729+t730+t731+t732+t748+t749+t750+t763+t764+t765+t769+t780+qdd1.*t25.*4.61e-2-qdd5.*t43.*1.844e-1-qdd2.*t90.*4.61e-2-qdd3.*t90.*4.61e-2;
et19 = qdd4.*t90.*(-4.61e-2)+qdd2.*t106.*4.61e-2+qdd3.*t106.*4.61e-2+qdd4.*t106.*4.61e-2+qdd1.*t121.*4.61e-2-qdd1.*t151.*2.305e-2-qdd1.*t199.*2.305e-2+t20.*t92.*4.61e-2+t21.*t92.*4.61e-2+t22.*t92.*4.61e-2-t20.*t108.*4.61e-2-t21.*t108.*4.61e-2-t22.*t108.*4.61e-2-qd1.*qd5.*t28.*9.22e-2+qd2.*qd5.*t47.*1.844e-1+qd3.*qd5.*t47.*1.844e-1;
et20 = qd4.*qd5.*t47.*1.844e-1+qd2.*qd3.*t92.*9.22e-2+qd2.*qd4.*t92.*9.22e-2+qd2.*qd5.*t92.*9.22e-2+qd3.*qd4.*t92.*9.22e-2+qd3.*qd5.*t92.*9.22e-2+qd4.*qd5.*t92.*9.22e-2-qd2.*qd3.*t108.*9.22e-2-qd2.*qd4.*t108.*9.22e-2+qd2.*qd5.*t108.*9.22e-2-qd3.*qd4.*t108.*9.22e-2+qd3.*qd5.*t108.*9.22e-2+qd4.*qd5.*t108.*9.22e-2+qd1.*qd2.*t155.*4.61e-2+qd1.*qd3.*t155.*4.61e-2+qd1.*qd4.*t155.*4.61e-2;
et21 = qd1.*qd5.*t155.*4.61e-2+qd1.*qd2.*t204.*4.61e-2+qd1.*qd3.*t204.*4.61e-2+qd1.*qd4.*t204.*4.61e-2-qd1.*qd5.*t204.*4.61e-2;
et22 = qdd2.*7.197082e-1+t256+t302+t348+t379+t382+t402+t442+t444+t475+t487+t505+t506+t509+t510+t516+t523+t524+t538+t539+t540+t541+t542+t543+t544+t568+t569+t570+t574+t575+t583+t588+t589+t590+t593+t621+t622+t624+t625+t627+t629+t630+t631+t632+t633+t634+t638+t643+t644+t645+t654+t662+t666+t667+t678+t685+t686+t696+t699+t701+t702+t709+t715+t723+t724+t728+t734+t736+t737+t741+t743+t744+t751+t758+t767+t774+t775+t785+t789+t794+t798+t800+t802+t805+t807+t808+qdd2.*t49.*5.64264e-2+qdd3.*t49.*2.82132e-2+qdd4.*t49.*2.82132e-2+qdd5.*t49.*2.82132e-2-qdd2.*t89.*5.64264e-2;
et23 = qdd3.*t89.*(-2.82132e-2)-qdd4.*t89.*2.82132e-2+qdd5.*t89.*2.82132e-2+t21.*t45.*2.82132e-2+t22.*t45.*2.82132e-2+t23.*t45.*2.82132e-2-t21.*t85.*2.82132e-2-t22.*t85.*2.82132e-2-t23.*t85.*2.82132e-2-t19.*t91.*2.82132e-2+t19.*t124.*2.82132e-2;
et24 = qd1.*qd5.*t30.*5.64264e-2+qd2.*qd3.*t45.*5.64264e-2+qd2.*qd4.*t45.*5.64264e-2+qd2.*qd5.*t45.*5.64264e-2+qd3.*qd4.*t45.*5.64264e-2+qd3.*qd5.*t45.*5.64264e-2+qd4.*qd5.*t45.*5.64264e-2-qd1.*qd5.*t64.*5.64264e-2-qd2.*qd3.*t85.*5.64264e-2-qd2.*qd4.*t85.*5.64264e-2;
et25 = qd2.*qd5.*t85.*5.64264e-2-qd3.*qd4.*t85.*5.64264e-2+qd3.*qd5.*t85.*5.64264e-2+qd4.*qd5.*t85.*5.64264e-2;
et26 = qdd5.*8.50084e-3-t74.*8.50084e-3-t75.*8.50084e-3-t77.*8.50084e-3-t444+t537+t593+t619+t620+t627+t636+t637-t638+t639+t660-t666-t697-t707-t708+t711+t712+t716+t725+t726+t733+t741-t754-t755-t759-t781+t797-t803+t804+t805-qdd2.*t5.*1.066754e-2-qdd3.*t5.*1.066754e-2-qdd4.*t5.*1.066754e-2;
et27 = qdd1.*t43.*(-8.50084e-3)-qdd1.*t59.*1.288956e-2-qdd1.*t105.*2.22202e-3+t9.*t19.*1.511158e-2+t19.*t28.*2.12521e-3-t20.*t28.*4.25042e-3-t21.*t28.*4.25042e-3-t22.*t28.*4.25042e-3+t19.*t135.*2.666885e-3+t19.*t203.*2.666885e-3;
et28 = qd1.*qd2.*t30.*(-5.64264e-2)-qd1.*qd2.*t44.*5.276606e-2-qd1.*qd3.*t44.*5.276606e-2+qd1.*qd2.*t47.*8.50084e-3+qd1.*qd3.*t47.*8.50084e-3+qd1.*qd4.*t47.*8.50084e-3+qd1.*qd2.*t60.*1.066754e-2+qd1.*qd3.*t60.*1.066754e-2+qd1.*qd4.*t60.*1.066754e-2+qd1.*qd2.*t64.*5.64264e-2;
et29 = qd1.*qd2.*t84.*5.276606e-2+qd1.*qd3.*t84.*5.276606e-2-qd1.*qd2.*t92.*4.25042e-3-qd1.*qd3.*t92.*4.25042e-3-qd1.*qd4.*t92.*4.25042e-3-qd1.*qd2.*t107.*1.066754e-2-qd1.*qd2.*t108.*4.25042e-3-qd1.*qd3.*t107.*1.066754e-2-qd1.*qd3.*t108.*4.25042e-3;
et30 = qd1.*qd4.*t107.*(-1.066754e-2)-qd1.*qd4.*t108.*4.25042e-3;
et31 = qdd5.*1.844e-1-t74.*1.844e-1-t75.*1.844e-1-t77.*1.844e-1+t171+t194+t236+t237+t238+t246+t252+t266+t267+t275+t278+t281+t283+t287+t326+t334+t364+t365+t373+t374+t375+t398+t399+t400+t403+t404+t405+t413+t414+t434+t449+t482+t497+t515+t517+t519+t520+t551+t552+t555+t604+t605+t606+t651+t676+t718+t761+t762+t770+t779-qdd1.*t43.*1.844e-1+t19.*t28.*4.61e-2-t20.*t28.*9.22e-2-t21.*t28.*9.22e-2-t22.*t28.*9.22e-2+qd1.*qd2.*t47.*1.844e-1+qd1.*qd3.*t47.*1.844e-1+qd1.*qd4.*t47.*1.844e-1;
et32 = qd1.*qd2.*t92.*(-9.22e-2)-qd1.*qd3.*t92.*9.22e-2-qd1.*qd4.*t92.*9.22e-2-qd1.*qd2.*t108.*9.22e-2-qd1.*qd3.*t108.*9.22e-2-qd1.*qd4.*t108.*9.22e-2;
mt1 = [qdd1,0.0,0.0,0.0,0.0,0.0,qdd1.*t26.*3.74544e-1-qd1.*qd2.*t2.*t6.*7.49088e-1,qdd2.*3.74544e-1+t256+t442,0.0,0.0,0.0,0.0,t94+qdd1.*t6.^2,-t126,0.0,0.0,0.0,0.0,-t94+qdd1.*t26,t126,0.0,0.0,0.0,0.0,0.0,qdd2,0.0,0.0,0.0,0.0,qdd1.*3.51035645e-1+t319+t378+t380+t488+t626+t670+t671+t760+t790+t791,t256+t379+t382+t442+t467+t475+t487+t530+t541+t667+t789,t381+t466+t467+t475+t479+t481+t668+t789,0.0,0.0,0.0,t51+t131+t132-(qdd1.*t80)./2.0,t273,t273,0.0,0.0,0.0,t51-t131-t132+t136,t235,t235,0.0,0.0,0.0,0.0,t14,t14,0.0,0.0,0.0];
mt2 = [qdd1.*3.77898855e-1+t319+t349+t378+t380+t418+t488+t626+t655+t656+t661+t670+t671+t713+t714+t760+t790+t791,t256+t348+t379+t382+t442+t467+t475+t487+t530+t541+t654+t667+t789,t381+t466+t467+t475+t479+t481+t654+t668+t789,0.0,0.0,0.0,et1+et2,t169+t182+t183+t205+t206+t240+t279+t306+t594-qdd2.*t39.*(1.53e+2./1.25e+2)-qdd3.*t39.*(1.53e+2./2.5e+2)-qdd4.*t39.*(1.53e+2./2.5e+2)-t21.*t31.*(1.53e+2./2.5e+2)-t22.*t31.*(1.53e+2./2.5e+2)+t19.*t70.*(1.53e+2./2.5e+2)-qd2.*qd3.*t31.*(1.53e+2./1.25e+2)-qd2.*qd4.*t31.*(1.53e+2./1.25e+2)-qd3.*qd4.*t31.*(1.53e+2./1.25e+2),t169+t170+t182+t183+t205+t206+t240+t242+t243+t279+t306+t347+t594];
mt3 = [t169+t170+t242+t243+t306+t347-qdd2.*t8.*5.723e-1-qdd3.*t8.*5.723e-1+t4.*t19.*2.8615e-1+t4.*t20.*5.723e-1+t4.*t21.*5.723e-1+t19.*t102.*2.8615e-1+qd2.*qd3.*t4.*1.1446,0.0,0.0,t51+t173+t174+t175-(qdd1.*t121)./2.0,t376,t376,t376,0.0,0.0,0.0,t36,t36,t36,0.0,0.0,t51+t249+t270+t271+t272,t344,t344,t344,0.0,0.0];
mt4 = [qdd1.*3.845921e-1+t173.*1.338649e-2+t174.*1.338649e-2+t175.*1.338649e-2+t319+t349+t378+t380+t418+t488+t507+t580+t591+t592+t599+t626+t640+t655+t656+t661+t663+t664+t665+t670+t671+t672+t673+t674+t680+t681+t682+t713+t714+t738+t739+t740+t760+t771+t772+t782+t787+t790+t791-qdd1.*t121.*6.693245e-3,qdd2.*7.1545778e-1+t256+t348+t379+t382+t397+t401+t442+t475+t487+t505+t506+t509+t510+t523+t524+t541+t543+t544+t583+t588+t589+t590+t624+t625+t634+t654+t662+t667+t678+t785+t789+t799];
mt5 = [qdd2.*3.4091378e-1+t381+t397+t401+t475+t479+t481+t505+t508+t523+t524+t543+t544+t583+t584+t587+t634+t654+t662+t668+t679+t785+t789+t799,qdd2.*1.338649e-2+qdd3.*1.338649e-2+t401+t483+t505+t508+t581+t582+t584+t587+t595+t596+t598+t662+t679+t786+t799,0.0,0.0,t139+t143+t172+t193+t210+t229+t230+t231+t244+t265+t274+t276+t277+t301+t303+t304+t305+t313+t314+t316+t317+t320+t321+t322+t323+t324+t330+t335+t337+t338+t339+t342+t358+t366+t368+t370+t371+t391+t392+t393+t394+t395+t396+t407+t408+t409+t425+t433+t435+t436+t437+t456+t457+t458+t471+t486+t500+t514+t518+t521+t546+t556+t557+t558+t563+t564+t565+t571+t572+t573+t576+t577+t600+t601+t602+t603+t615+t616+t617+t618+t623+t650+t706+t722+t729+t730+t731+t732+t748+t749+t750+t763+t764+t765+t769+t780];
mt6 = [t138+t191+t192+t195+t196+t197+t223+t224+t225+t226+t227+t228+t239+t251+t259+t260+t261+t263+t264+t268+t269+t275+t278+t290+t308+t309+t310+t311+t312+t315+t327+t328+t329+t332+t333+t336+t343+t352+t354+t355+t361+t362+t388+t389+t390+t416+t419+t428+t430+t431+t434+t450+t451+t452+t455+t468+t469+t470+t474+t498+t499+t553+t554+t562+t567+t579+t675+t717+t746+t788,t194+t239+t251+t263+t264+t268+t269+t278+t281+t308+t309+t310+t311+t312+t315+t326+t328+t331+t336+t343+t361+t362+t383+t416+t428+t430+t431+t434+t453+t455+t468+t469+t470+t474+t482+t498+t499+t553+t554+t562+t579+t614+t675+t717+t746+t788,t194+t239+t251+t266+t267+t278+t281+t326+t328+t331+t336+t364+t383+t398+t399+t400+t426+t453+t455+t468+t472+t473+t482+t489+t490+t493+t562+t614+t676+t717+t747+t788,t171+t194+t236+t237+t238+t246+t252+t266+t267+t275+t278+t281+t283+t287+t326+t334+t364+t365+t373+t374+t375+t398+t399+t400+t403+t404+t405+t413+t414+t434+t449+t482+t497+t515+t517+t519+t520+t551+t552+t555+t604+t605+t606+t651+t676+t718+t770+t779];
mt7 = [0.0,t53+t96-t115-t148-t149-t150+t162+t164+t165+t166+t167+t168+t187+t188+t189+t207+t208+t209-t215-t218+t219-t220+t221+t222-t253-t254-t255+t280+t298+t299+t300+t438+t439+t440+t441-t465+t501+t502+t503-t504-t529,t809,t809,t809,-t74-t75-t77-t127+t128-t129-t130-t159-t160-t161-t212-t213-t214+t607+t608,0.0,t51+t249+t270+t271+t272-qdd5.*t43+qd2.*qd5.*t47+qd3.*qd5.*t47+qd4.*qd5.*t47,t776,t776,t776,qdd5-qdd1.*t43+qd1.*qd2.*t47+qd1.*qd3.*t47+qd1.*qd4.*t47,0.0];
mt8 = [t53+t115+t148+t149+t150-t162-t164-t165-t166-t167-t168-t187-t188-t189-t207-t208-t209+t215+t218-t219+t220-t221-t222+t253+t254+t255+t280+t298+t299+t300-t438-t439-t440-t441+t465-t501-t502-t503+t504+t529-(qdd1.*t25)./4.0,t810,t810,t810,t74+t75+t77+t127-t128+t129+t130+t159+t160+t161+t212+t213+t214+t566+t635,0.0,et3+et4+et5+et6+et7+et8+et9+et10+et11+et12+et13+et14+et15+et16+et17,et22+et23+et24+et25];
mt9 = [qdd2.*3.451642e-1+t302+t381+t402+t475+t479+t481+t505+t508+t516+t523+t524+t537+t538+t539+t540+t542+t543+t544+t568+t569+t570+t574+t575+t583+t584+t587+t593+t621+t622+t629+t630+t631+t632+t633+t634+t636+t637+t638+t643+t644+t645+t654+t662+t666+t668+t669+t679+t685+t686+t696+t699+t701+t702+t707+t708+t709+t715+t723+t724+t728+t733+t734+t736+t737+t741+t743+t744+t751+t758+t767+t774+t775+t781+t785+t789+t794+t798+t800+t802+t805+t807+t808];
mt10 = [qdd2.*1.763691e-2+qdd3.*1.763691e-2+t402+t483+t505+t508+t516+t537+t538+t539+t540+t542+t568+t569+t570+t581+t582+t584+t587+t593+t595+t596+t598+t619+t620+t636+t637+t638+t643+t645+t660+t662+t669+t679+t696+t697+t707+t708+t709+t711+t712+t715+t716-t725-t726+t733+t734+t743+t744+t754+t755+t758+t759+t781+t786+t797+t798+t800+t803+t805+t807+t808,et26+et27+et28+et29+et30,0.0,et18+et19+et20+et21];
mt11 = [t117+t118+t119+t138+t191+t192+t195+t196+t197+t200+t201+t202+t223+t224+t225+t226+t227+t228+t232+t233+t234+t239+t251+t259+t260+t261+t263+t264+t268+t269+t275+t278+t290+t297+t308+t309+t310+t311+t312+t315+t327+t328+t329+t332+t333+t336+t343+t352+t354+t355+t361+t362+t369+t388+t389+t390+t416+t419+t424+t428+t430+t431+t434+t450+t451+t452+t455+t461+t462+t468+t469+t470+t474+t498+t499+t553+t554+t562+t567+t579+t649+t675+t717+t746+t762+t777+t788,t117+t118+t119+t194+t200+t201+t202+t232+t233+t234+t239+t251+t263+t264+t268+t269+t278+t281+t297+t308+t309+t310+t311+t312+t315+t326+t328+t331+t336+t343+t361+t362+t369+t383+t416+t424+t428+t430+t431+t434+t453+t455+t461+t462+t468+t469+t470+t474+t482+t498+t499+t553+t554+t562+t579+t614+t649+t675+t717+t746+t762+t777+t788];
mt12 = [t117+t118+t119+t194+t200+t201+t202+t232+t233+t234+t239+t251+t266+t267+t278+t281+t297+t326+t328+t331+t336+t364+t369+t383+t398+t399+t400+t424+t426+t453+t455+t461+t462+t468+t472+t473+t482+t489+t490+t493+t562+t614+t649+t676+t717+t747+t762+t777+t788,et31+et32,0.0,0.0,0.0,0.0,0.0,0.0,0.0,0.0,0.0,0.0,0.0,0.0,0.0,0.0,0.0,0.0,0.0,0.0,0.0];
Y = reshape([mt1,mt2,mt3,mt4,mt5,mt6,mt7,mt8,mt9,mt10,mt11,mt12],6,24);
end
